simulink model "mdlref_depgraph"  (Simulink 6.0)
settings: Solver=ode3  SolverMode=SingleTasking  StartTime=0.0  StopTime=2*24*60*60  FixedStep=60  RelTol=1e-3  AbsTol=1e-6
PreLoadFcn:
  | thermdat
settings Model: Creator=The MathWorks Inc.  LastModifiedBy=batserve  ExtModeTrigMode=oneshot  ExtModeArmWhenConnect=off  ExtModeAutoUpdateStatusClock=off
settings DataIOCC: ExternalInput=[]  InitialState=[]  LimitDataPoints=off  SaveOutput=off  SaveTime=off
settings OptimizationCC: BlockReduction=off  BooleanDataType=off  InlineParams=on
settings DebuggingCC: CheckExecutionContextPreStartOutputMsg=on  CheckExecutionContextRuntimeOutputMsg=on  SignalResolutionControl=UseLocalSettings  SolverPrmCheckMsg=none  DiscreteInheritContinuousMsg=none  IntegerOverflowMsg=none
settings HardwareCC: TargetUnknown=on
settings ModelReferenceCC: UpdateModelReferenceTargets=IfOutOfDate

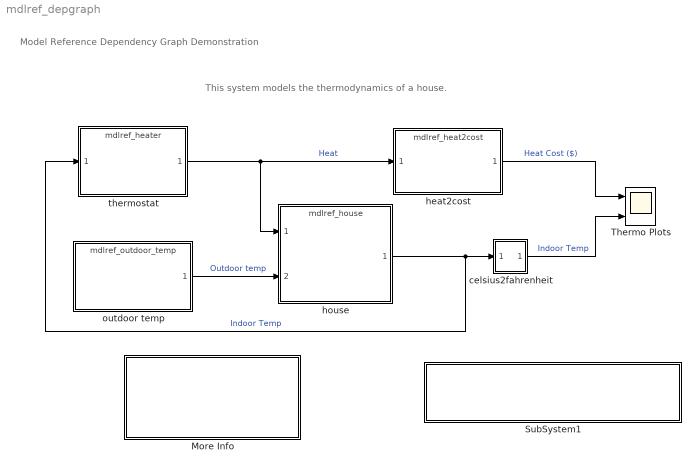
== system mdlref_depgraph ==
  note: Model Reference Dependency Graph Demonstration
  note: This system models the thermodynamics of a house.
  More Info : Subsystem  PropExecContextAcrossSSBoundary=on
      settings: OpenFcn="mFileName = 'mdlref_depgraph_demo'; htmlName      = 'mdlref_depgraph_demo.html';fullPath      = which(mFileName); dirPath       = fileparts(fullPath);fullHTMLPath  = fullfile(dirPath,htmlName);web(fullHTMLPath,'-helpbrowser')"
      mask Display: disp('Double click here \nfor a step-by-step\ntutorial on this model')
  SubSystem1 : Subsystem  PropExecContextAcrossSSBoundary=on
      settings: OpenFcn=|
      | mdlName= get_param(bdroot(gcbh),'name');
      | view_mdlrefs(mdlName);
      mask Display: disp('Double click here to view \n Model Reference dependency graph');
  Thermo Plots : Scope  NumInputPorts=2
      settings: TickLabels=on  TimeRange=200000  YMin=0~60  YMax=40~80
  celsius2fahrenheit : Subsystem  PropExecContextAcrossSSBoundary=on
      mask Type: CelsiusToFahrenheit
      mask Description:
      | Conversion from degrees Celsius to degrees Fahrenheit.
      | 
      | F=9/5*C+32
      mask Help: This block converts from degrees Celsius to degrees Fahrenheit.
      mask Display: disp('C2F')
  heat2cost : ModelReference  ModelName=mdlref_heat2cost  ModelReferenceVersion=1.7  CopyOfModelName=mdlref_heat2cost
  house : ModelReference  ModelName=mdlref_house  ModelReferenceVersion=1.7  CopyOfModelName=mdlref_house
  outdoor temp : ModelReference  ModelName=mdlref_outdoor_temp  ModelReferenceVersion=1.13  CopyOfModelName=mdlref_outdoor_temp
  thermostat : ModelReference  ModelName=mdlref_heater  ModelReferenceVersion=1.17  CopyOfModelName=mdlref_heater
  wires:
  thermostat/1 -> house/1, heat2cost/1  "Heat"
  house/1 -> celsius2fahrenheit/1(Celsius in), thermostat/1  "Indoor Temp"
  outdoor temp/1 -> house/2  "Outdoor temp"
  heat2cost/1 -> Thermo Plots/1  "Heat Cost ($)"
  celsius2fahrenheit/1(Fahrenheit out) -> Thermo Plots/2  "Indoor Temp"

== system mdlref_depgraph/More Info ==

== system mdlref_depgraph/SubSystem1 ==

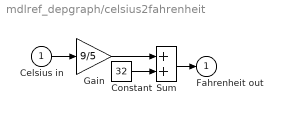
== system mdlref_depgraph/celsius2fahrenheit ==
  Celsius in : Inport  Port=1  LatchInput=off
  Constant : Constant  Value=32
  Gain : Gain  Gain=9/5  SaturateOnIntegerOverflow=on
  Sum : Sum  SaturateOnIntegerOverflow=on  InputSameDT=on
  Fahrenheit out : Outport  InitialOutput=0
  wires:
  Celsius in/1 -> Gain/1
  Gain/1 -> Sum/1
  Sum/1 -> Fahrenheit out/1
  Constant/1 -> Sum/2
